simulink model "p2"  (R2023a)
settings: Solver=VariableStepAuto  StartTime=0.0  StopTime=10.0  RelTol=1e-3
settings Model: Creator=ssata  LastModifiedBy=ssata

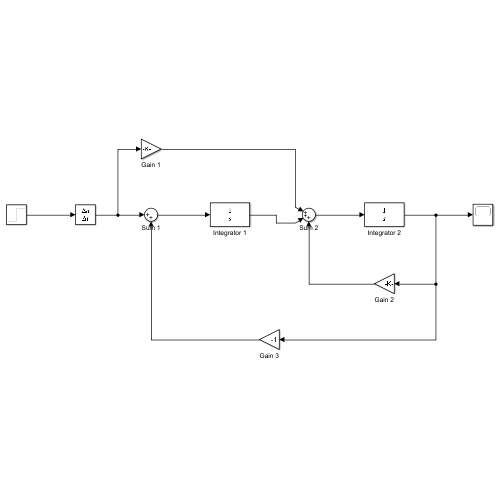
[thumbnail: Simulink's stored preview of the top-level diagram]
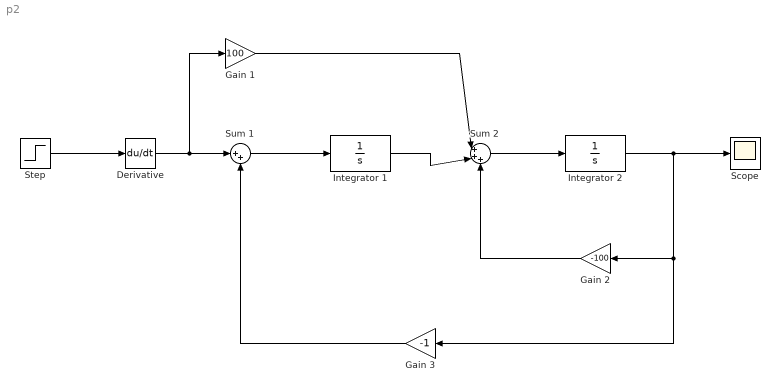
== system p2 ==
  Derivative : Derivative
  Gain 1 : Gain  Gain=100
  Gain 2 : Gain  Gain=-100
  Gain 3 : Gain  Gain=-1
  Integrator 1 : TransferFcn  Denominator=[1 0]
  Integrator 2 : TransferFcn  Denominator=[1 0]
  Scope : Scope
  Step : Step  Time=0.001  SampleTime=0
  Sum 1 : Sum  Inputs=|++
  Sum 2 : Sum  Inputs=|+++
  wires:
  Step/1 -> Derivative/1
  Derivative/1 -> Gain 1/1, Sum 1/1
  Gain 1/1 -> Sum 2/1
  Integrator 1/1 -> Sum 2/2
  Sum 1/1 -> Integrator 1/1
  Gain 3/1 -> Sum 1/2
  Gain 2/1 -> Sum 2/3
  Integrator 2/1 -> Gain 3/1, Gain 2/1, Scope/1
  Sum 2/1 -> Integrator 2/1
